simulink model "E040S1_R2_transfer_drain_iqcot_20260630"  (R2024b)
settings: Solver=VariableStepAuto  StartTime=0.0  StopTime=0.52e-3  MaxStep=5e-9  RelTol=1e-3
undefined symbols (not defined in the file): A_init, A_lower, A_upper, Cout, DCR_L1, DCR_L2, DCR_L3, DCR_L4, E040_Calibration_Enable, E040_Current_Deadband, E040_Current_Limit_A, E040_Disabled_Phase_Drain_Timeout, E040_Dwell_Time, E040_Fallback_K_T, E040_I_Shed_Low, E040_IL_Sense_Gain1, E040_IL_Sense_Gain2, E040_IL_Sense_Gain3, E040_IL_Sense_Gain4, E040_K_T, E040_LoadStep_Time, E040_Max_Transfer_Ton_Trim, E040_Min_Scale, E040_Order_Relock_Window, E040_Post_Reentry_Shed_Delay, E040_Post_Shed_AS_Delay, E040_Remaining_Phase_Current_Limit, E040_Residual_Current_Threshold, E040_Sense_Confidence, E040_Severe_Overshoot_Band, E040_Shed_Commit_Boundary_Policy, E040_Shed_Fallback_Enable, E040_Shed_Transfer_Rate, E040_Shed_Transfer_Window, E040_Shed_Undershoot_Budget, E040_T_Trim_Max, E040_TonDiff_Enable, E040_V_Error_Budget, E040_V_Error_Hard_Limit, E040_Variant_Mode, E040_Vref, ESR_C, IdealIQCOT_Enable, IL_adc_counts_per_A, IL_pk_limit_adc_neg, IL_pk_limit_adc_pos, Iload_final, Iload_initial, Iph, Iqcot_enable, kappa_cmd, Kiqcot, Kvc_iqcot, L, Lambda0_iqcot, Lambda_m2, rho_cmd, Ri_iqcot, t_load_step, Tblank ... (+15)
libraries: simulink x29, spsCurrentMeasurementLib x8, spsMosfetLib x8, spsSeriesRLCBranchLib x5, spsVoltageMeasurementLib x5, spsDCVoltageSourceLib x4, spsControlledCurrentSourceLib x1, spsGroundLib x1, spspowerguiLib x1
(part 2 of 2)

== system E040S1_R2_transfer_drain_iqcot_20260630/OnDelay ==
  u : Inport
  Compare To Constant : simulink/Logic and Bit Operations/Compare To Constant  relop=>=  const=Tdead  OutDataTypeStr=boolean
  Data Type Conversion : DataTypeConversion  OutDataTypeStr=double  SaturateOnIntegerOverflow=off  RndMeth=Floor
  Integrator : Integrator  ExternalReset=level
  Logical Operator : Logic  Operator=NOT  AllPortsSameDT=off  OutDataTypeStr=boolean
  y : Outport
  wires:
  u/1 -> Data Type Conversion/1, Logical Operator/1
  Logical Operator/1 -> Integrator/2
  Data Type Conversion/1 -> Integrator/1
  Integrator/1 -> Compare To Constant/1
  Compare To Constant/1 -> y/1

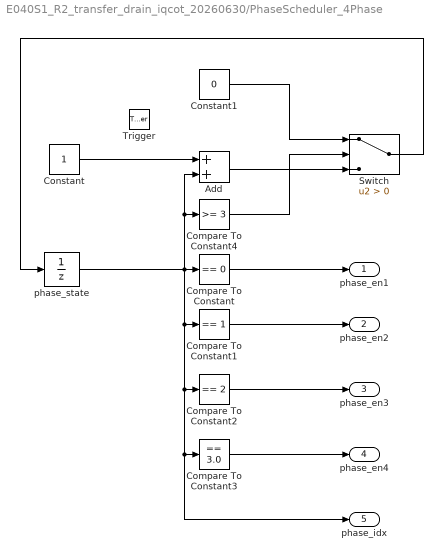
== system E040S1_R2_transfer_drain_iqcot_20260630/PhaseScheduler_4Phase ==
  Trigger : TriggerPort  VariantControl=(inherit)
  Add : Sum
  Compare To Constant : simulink/Logic and Bit Operations/Compare To Constant  relop===  const=0  OutDataTypeStr=boolean
  Compare To Constant1 : simulink/Logic and Bit Operations/Compare To Constant  relop===  const=1  OutDataTypeStr=boolean
  Compare To Constant2 : simulink/Logic and Bit Operations/Compare To Constant  relop===  const=2  OutDataTypeStr=boolean
  Compare To Constant3 : simulink/Logic and Bit Operations/Compare To Constant  relop===  const=3.0  OutDataTypeStr=boolean
  Compare To Constant4 : simulink/Logic and Bit Operations/Compare To Constant  relop=>=  const=3  OutDataTypeStr=boolean
  Constant : Constant
  Constant1 : Constant  Value=0
  Switch : Switch  Criteria=u2 > Threshold  SaturateOnIntegerOverflow=off  InputSameDT=off
  phase_state : UnitDelay  SampleTime=-1  HasFrameUpgradeWarning=on
  phase_en1 : Outport
  phase_en2 : Outport  Port=2
  phase_en3 : Outport  Port=3
  phase_en4 : Outport  Port=4
  phase_idx : Outport  Port=5
  wires:
  phase_state/1 -> phase_idx/1, Compare To Constant3/1, Compare To Constant2/1, Compare To Constant1/1, Compare To Constant/1, Compare To Constant4/1, Add/2
  Compare To Constant/1 -> phase_en1/1
  Compare To Constant1/1 -> phase_en2/1
  Compare To Constant2/1 -> phase_en3/1
  Compare To Constant3/1 -> phase_en4/1
  Constant/1 -> Add/1
  Add/1 -> Switch/3
  Compare To Constant4/1 -> Switch/2
  Constant1/1 -> Switch/1
  Switch/1 -> phase_state/1

== system E040S1_R2_transfer_drain_iqcot_20260630/GateDriver_1Phase1/OnDelay ==
  u : Inport
  Compare To Constant : simulink/Logic and Bit Operations/Compare To Constant  relop=>=  const=Tdead  OutDataTypeStr=boolean
  Data Type Conversion : DataTypeConversion  OutDataTypeStr=double  SaturateOnIntegerOverflow=off  RndMeth=Floor
  Integrator : Integrator  ExternalReset=level
  Logical Operator : Logic  Operator=NOT  AllPortsSameDT=off  OutDataTypeStr=boolean
  y : Outport
  wires:
  u/1 -> Data Type Conversion/1, Logical Operator/1
  Logical Operator/1 -> Integrator/2
  Data Type Conversion/1 -> Integrator/1
  Integrator/1 -> Compare To Constant/1
  Compare To Constant/1 -> y/1

== system E040S1_R2_transfer_drain_iqcot_20260630/GateDriver_1Phase1/OnDelay1 ==
  u : Inport
  Compare To Constant : simulink/Logic and Bit Operations/Compare To Constant  relop=>=  const=Tdead  OutDataTypeStr=boolean
  Data Type Conversion : DataTypeConversion  OutDataTypeStr=double  SaturateOnIntegerOverflow=off  RndMeth=Floor
  Integrator : Integrator  ExternalReset=level
  Logical Operator : Logic  Operator=NOT  AllPortsSameDT=off  OutDataTypeStr=boolean
  y : Outport
  wires:
  u/1 -> Data Type Conversion/1, Logical Operator/1
  Logical Operator/1 -> Integrator/2
  Data Type Conversion/1 -> Integrator/1
  Integrator/1 -> Compare To Constant/1
  Compare To Constant/1 -> y/1

== system E040S1_R2_transfer_drain_iqcot_20260630/GateDriver_1Phase2/OnDelay ==
  u : Inport
  Compare To Constant : simulink/Logic and Bit Operations/Compare To Constant  relop=>=  const=Tdead  OutDataTypeStr=boolean
  Data Type Conversion : DataTypeConversion  OutDataTypeStr=double  SaturateOnIntegerOverflow=off  RndMeth=Floor
  Integrator : Integrator  ExternalReset=level
  Logical Operator : Logic  Operator=NOT  AllPortsSameDT=off  OutDataTypeStr=boolean
  y : Outport
  wires:
  u/1 -> Data Type Conversion/1, Logical Operator/1
  Logical Operator/1 -> Integrator/2
  Data Type Conversion/1 -> Integrator/1
  Integrator/1 -> Compare To Constant/1
  Compare To Constant/1 -> y/1

== system E040S1_R2_transfer_drain_iqcot_20260630/GateDriver_1Phase2/OnDelay1 ==
  u : Inport
  Compare To Constant : simulink/Logic and Bit Operations/Compare To Constant  relop=>=  const=Tdead  OutDataTypeStr=boolean
  Data Type Conversion : DataTypeConversion  OutDataTypeStr=double  SaturateOnIntegerOverflow=off  RndMeth=Floor
  Integrator : Integrator  ExternalReset=level
  Logical Operator : Logic  Operator=NOT  AllPortsSameDT=off  OutDataTypeStr=boolean
  y : Outport
  wires:
  u/1 -> Data Type Conversion/1, Logical Operator/1
  Logical Operator/1 -> Integrator/2
  Data Type Conversion/1 -> Integrator/1
  Integrator/1 -> Compare To Constant/1
  Compare To Constant/1 -> y/1

== system E040S1_R2_transfer_drain_iqcot_20260630/GateDriver_1Phase3/OnDelay ==
  u : Inport
  Compare To Constant : simulink/Logic and Bit Operations/Compare To Constant  relop=>=  const=Tdead  OutDataTypeStr=boolean
  Data Type Conversion : DataTypeConversion  OutDataTypeStr=double  SaturateOnIntegerOverflow=off  RndMeth=Floor
  Integrator : Integrator  ExternalReset=level
  Logical Operator : Logic  Operator=NOT  AllPortsSameDT=off  OutDataTypeStr=boolean
  y : Outport
  wires:
  u/1 -> Data Type Conversion/1, Logical Operator/1
  Logical Operator/1 -> Integrator/2
  Data Type Conversion/1 -> Integrator/1
  Integrator/1 -> Compare To Constant/1
  Compare To Constant/1 -> y/1

== system E040S1_R2_transfer_drain_iqcot_20260630/GateDriver_1Phase3/OnDelay1 ==
  u : Inport
  Compare To Constant : simulink/Logic and Bit Operations/Compare To Constant  relop=>=  const=Tdead  OutDataTypeStr=boolean
  Data Type Conversion : DataTypeConversion  OutDataTypeStr=double  SaturateOnIntegerOverflow=off  RndMeth=Floor
  Integrator : Integrator  ExternalReset=level
  Logical Operator : Logic  Operator=NOT  AllPortsSameDT=off  OutDataTypeStr=boolean
  y : Outport
  wires:
  u/1 -> Data Type Conversion/1, Logical Operator/1
  Logical Operator/1 -> Integrator/2
  Data Type Conversion/1 -> Integrator/1
  Integrator/1 -> Compare To Constant/1
  Compare To Constant/1 -> y/1

== system E040S1_R2_transfer_drain_iqcot_20260630/GateDriver_1Phase4/OnDelay ==
  u : Inport
  Compare To Constant : simulink/Logic and Bit Operations/Compare To Constant  relop=>=  const=Tdead  OutDataTypeStr=boolean
  Data Type Conversion : DataTypeConversion  OutDataTypeStr=double  SaturateOnIntegerOverflow=off  RndMeth=Floor
  Integrator : Integrator  ExternalReset=level
  Logical Operator : Logic  Operator=NOT  AllPortsSameDT=off  OutDataTypeStr=boolean
  y : Outport
  wires:
  u/1 -> Data Type Conversion/1, Logical Operator/1
  Logical Operator/1 -> Integrator/2
  Data Type Conversion/1 -> Integrator/1
  Integrator/1 -> Compare To Constant/1
  Compare To Constant/1 -> y/1

== system E040S1_R2_transfer_drain_iqcot_20260630/GateDriver_1Phase4/OnDelay1 ==
  u : Inport
  Compare To Constant : simulink/Logic and Bit Operations/Compare To Constant  relop=>=  const=Tdead  OutDataTypeStr=boolean
  Data Type Conversion : DataTypeConversion  OutDataTypeStr=double  SaturateOnIntegerOverflow=off  RndMeth=Floor
  Integrator : Integrator  ExternalReset=level
  Logical Operator : Logic  Operator=NOT  AllPortsSameDT=off  OutDataTypeStr=boolean
  y : Outport
  wires:
  u/1 -> Data Type Conversion/1, Logical Operator/1
  Logical Operator/1 -> Integrator/2
  Data Type Conversion/1 -> Integrator/1
  Integrator/1 -> Compare To Constant/1
  Compare To Constant/1 -> y/1

== matlab function E040S1_R2_transfer_drain_iqcot_20260630/E040_S1_StagedShedSupervisor ==
  data: req1 input boolean; req1o output boolean; req2 input boolean; req3 input boolean; req4 input boolean; ton1 input double; ton2 input double; ton3 input double; ton4 input double; il1 input double; il2 input double; il3 input double; il4 input double; vout input double; iload input double; t input double; t_step input double; variant_mode input double; I_shed_low input double; dwell_time input double; post_reentry_shed_delay input double; Vref input double; severe_overshoot_band input double; current_limit_A input double; TonDiff_enable input double; K_T input double; fallback_K_T input double; T_trim_Max input double; current_deadband input double; sense_confidence input double; calibration_enable input double; Verr_budget input double; Verr_hard input double; min_scale input double; residual_current_threshold input double; order_relock_window input double; shed_transfer_rate input double; shed_transfer_window input double; max_transfer_Ton_trim input double; remaining_phase_current_limit_guard input double; disabled_phase_drain_timeout input double; shed_undershoot_budget input double; post_shed_aS_delay input double; shed_fallback_enable input double; shed_commit_boundary_policy input double; req2o output boolean; req3o output boolean; req4o output boolean; ton1o output double; ton2o output double; ton3o output double; ton4o output double; active_phase_set output double; N_active output double; phase_shed_request output double; phase_shed_accept output double; phase_shed_reject output double; phase_add_request output double; shed_state output double; shed_lockout_state output double; residual_current_i output double; residual_current_threshold_o output double; residual_current_check output double; dwell_timer output double; post_reentry_shed_delay_timer output double; protect_state output double; reentry_state output double; balance_recovery_state output double; sense_confidence_o output double; calibration_enable_o output double; a_S_mode output double; fallback_count_o output double; guard_clamp_count_o output double; trim1 output double; trim2 output double; trim3 output double; trim4 output double; REQ_accept1 output boolean; REQ_accept2 output boolean; REQ_accept3 output boolean; REQ_accept4 output boolean; REQ_reject_reason output double; logical_slot output double; physical_phase_selected output double; phase_shed_reject_reason output double; order_relock_state output double; order_relock_window_done output double; phase_order_error_rate_window output double; a_S_enable_after_shed output double; current_limit_hit output double; shed_transfer_progress output double; disabled_phase_current_sum output double; commit_armed output double; commit_done output double; shed_commit_count output double; fallback_4ph_triggered output double; fallback_reason output double; fallback_4ph_count output double; residual_current_phase2_A output double; residual_current_phase4_A output double; Ton_trim_usage output double; Lambda_trim_usage output double; phase_gate_enable1 output double; phase_gate_enable2 output double; phase_gate_enable3 output double; phase_gate_enable4 output double
function [req1o,req2o,req3o,req4o,ton1o,ton2o,ton3o,ton4o,active_phase_set,N_active,phase_shed_request,phase_shed_accept,phase_shed_reject,phase_add_request,shed_state,shed_lockout_state,residual_current_i,residual_current_threshold_o,residual_current_check,dwell_timer,post_reentry_shed_delay_timer,protect_state,reentry_state,balance_recovery_state,sense_confidence_o,calibration_enable_o,a_S_mode,fallback_count_o,guard_clamp_count_o,trim1,trim2,trim3,trim4,REQ_accept1,REQ_accept2,REQ_accept3,REQ_accept4,REQ_reject_reason,logical_slot,physical_phase_selected,phase_shed_reject_reason,order_relock_state,order_relock_window_done,phase_order_error_rate_window,a_S_enable_after_shed,current_limit_hit,shed_transfer_progress,disabled_phase_current_sum,commit_armed,commit_done,shed_commit_count,fallback_4ph_triggered,fallback_reason,fallback_4ph_count,residual_current_phase2_A,residual_current_phase4_A,Ton_trim_usage,Lambda_trim_usage,phase_gate_enable1,phase_gate_enable2,phase_gate_enable3,phase_gate_enable4] = e040_s1_supervisor(req1,req2,req3,req4,ton1,ton2,ton3,ton4,il1,il2,il3,il4,vout,iload,t,t_step,variant_mode,I_shed_low,dwell_time,post_reentry_shed_delay,Vref,severe_overshoot_band,current_limit_A,TonDiff_enable,K_T,fallback_K_T,T_trim_Max,current_deadband,sense_confidence,calibration_enable,Verr_budget,Verr_hard,min_scale,residual_current_threshold,order_relock_window,shed_transfer_rate,shed_transfer_window,max_transfer_Ton_trim,remaining_phase_current_limit_guard,disabled_phase_drain_timeout,shed_undershoot_budget,post_shed_aS_delay,shed_fallback_enable,shed_commit_boundary_policy)
%#codegen
req = [req1, req2, req3, req4] > 0.5;
tons = [ton1, ton2, ton3, ton4];
ils = [il1, il2, il3, il4];
phase_add_request = 0.0;
protect_state = 0.0;
reentry_state = 1.0;
sense_confidence_o = sense_confidence;
calibration_enable_o = calibration_enable;
residual_current_threshold_o = residual_current_threshold;
residual_current_phase2_A = il2;
residual_current_phase4_A = il4;
residual_current_i = [0.0, il2, 0.0, il4];
disabled_phase_current_sum = abs(il2) + abs(il4);
residual_ok = (residual_current_threshold > 0.0) && (abs(il2) <= residual_current_threshold) && (abs(il4) <= residual_current_threshold);
residual_current_check = double(residual_ok);
age = max(0.0, t - t_step);
request_active = (variant_mode > 0.5) && (iload < I_shed_low) && (t >= t_step);
phase_shed_request = double(request_active);
if request_active
    dwell_timer = age;
    post_reentry_shed_delay_timer = age;
else
    dwell_timer = 0.0;
    post_reentry_shed_delay_timer = 0.0;
end
transfer_window = max(shed_transfer_window, 1.0e-9);
drain_timeout = max(disabled_phase_drain_timeout, 0.0);
drain_deadline_age = transfer_window + drain_timeout;
post_transfer_age = max(0.0, age - transfer_window);
shed_transfer_progress = 0.0;
if request_active
    shed_transfer_progress = min(max(age / transfer_window, 0.0), 1.0);
end
phase2_drained = request_active && (variant_mode >= 2.0) && (shed_transfer_progress >= 0.5) && (residual_current_threshold > 0.0) && (abs(il2) <= residual_current_threshold);
phase4_drained = request_active && (variant_mode >= 2.0) && (shed_transfer_progress >= 0.5) && (residual_current_threshold > 0.0) && (abs(il4) <= residual_current_threshold);
current_limit_hit = double((current_limit_A > 0.0) && (max(abs(ils)) >= current_limit_A));
remaining_peak = max(abs(il1), abs(il3));
remaining_headroom_ok = (remaining_phase_current_limit_guard <= 0.0) || (remaining_peak < remaining_phase_current_limit_guard);
voltage_ok = (vout >= (Vref - shed_undershoot_budget)) && (vout <= (Vref + severe_overshoot_band));
drain_time_ok = (drain_timeout <= 0.0) || (age <= drain_deadline_age);
drain_timeout_fail = request_active && (variant_mode >= 3.0) && (age > drain_deadline_age) && ~residual_ok;
hard_guard_fail = request_active && (shed_fallback_enable > 0.5) && ((vout < Vref - shed_undershoot_budget) || current_limit_hit > 0.5 || ~remaining_headroom_ok || drain_timeout_fail);
fallback_4ph_triggered = double(hard_guard_fail);
fallback_4ph_count = fallback_4ph_triggered;
fallback_count_o = fallback_4ph_triggered;
fallback_reason = 0.0;
if hard_guard_fail
    if vout < Vref - shed_undershoot_budget
        fallback_reason = 1.0;
    elseif current_limit_hit > 0.5
        fallback_reason = 2.0;
    elseif drain_timeout_fail
        fallback_reason = 3.0;
    elseif ~remaining_headroom_ok
        fallback_reason = 5.0;
    else
        fallback_reason = 6.0;
    end
end
immediate_shed = request_active && (variant_mode >= 1.0) && (variant_mode < 2.0);
allow_commit_variant = variant_mode >= 3.0;
commit_ready = request_active && allow_commit_variant && (age >= transfer_window) && residual_ok && remaining_headroom_ok && voltage_ok && drain_time_ok && ~hard_guard_fail;
commit_hold = request_active && allow_commit_variant && (age >= transfer_window) && remaining_headroom_ok && voltage_ok && ~hard_guard_fail;
commit_armed = double(commit_ready || commit_hold || immediate_shed);
commit_done = double(commit_hold || immediate_shed);
shed_commit_count = commit_done;
commit_age = post_transfer_age;
order_relock_done = (commit_done > 0.5) && (commit_age >= max(order_relock_window, 0.0));
order_relock_window_done = double(order_relock_done);
a_S_enable_after_shed = double((variant_mode >= 4.0) && (TonDiff_enable > 0.5) && (commit_done > 0.5) && order_relock_done && residual_ok && voltage_ok && (commit_age >= max(post_shed_aS_delay, 0.0)));
balance_enable = a_S_enable_after_shed > 0.5;
phase_shed_accept = commit_done;
phase_shed_reject = double(request_active && commit_done < 0.5);
phase_shed_reject_reason = 0.0;
if phase_shed_reject > 0.5
    if hard_guard_fail
        phase_shed_reject_reason = fallback_reason;
    elseif age < transfer_window
        phase_shed_reject_reason = 2.0;
    elseif ~residual_ok
        phase_shed_reject_reason = 3.0;
    elseif ~remaining_headroom_ok
        phase_shed_reject_reason = 5.0;
    else
        phase_shed_reject_reason = 1.0;
    end
end
if ~request_active
    shed_state = 0.0;
    shed_lockout_state = 0.0;
    order_relock_state = 0.0;
elseif hard_guard_fail
    shed_state = 9.0;
    shed_lockout_state = 1.0;
    order_relock_state = 0.0;
elseif age < 1.0e-7
    shed_state = 1.0;
    shed_lockout_state = 0.0;
    order_relock_state = 1.0;
elseif age < transfer_window
    shed_state = 2.0;
    shed_lockout_state = 0.0;
    order_relock_state = 1.0;
elseif immediate_shed
    shed_state = 5.0;
    shed_lockout_state = 0.0;
    order_relock_state = 2.0;
elseif age >= transfer_window && (~residual_ok || ~remaining_headroom_ok || ~voltage_ok)
    shed_state = 3.0;
    shed_lockout_state = 0.0;
    order_relock_state = 1.0;
elseif variant_mode < 3.0
    shed_state = 3.0;
    shed_lockout_state = 0.0;
    order_relock_state = 1.0;
elseif commit_done < 0.5
    shed_state = 4.0;
    shed_lockout_state = 0.0;
    order_relock_state = 1.0;
elseif commit_age < 5.0e-8
    shed_state = 5.0;
    shed_lockout_state = 0.0;
    order_relock_state = 2.0;
elseif ~order_relock_done
    shed_state = 6.0;
    shed_lockout_state = 0.0;
    order_relock_state = 2.0;
elseif balance_enable
    shed_state = 7.0;
    shed_lockout_state = 0.0;
    order_relock_state = 3.0;
else
    shed_state = 8.0;
    shed_lockout_state = 0.0;
    order_relock_state = 3.0;
end
trim = [0.0, 0.0, 0.0, 0.0];
if request_active && ~hard_guard_fail && (variant_mode >= 2.0) && (commit_done < 0.5)
    p = shed_transfer_progress;
    transfer_trim = min(max_transfer_Ton_trim, T_trim_Max);
    if transfer_trim < 0.0
        transfer_trim = 0.0;
    end
    trim = [p * transfer_trim, -p * transfer_trim, p * transfer_trim, -p * transfer_trim];
end
REQ_reject_reason = 0.0;
if hard_guard_fail
    active_phase_set = [1.0, 1.0, 1.0, 1.0];
    N_active = 4.0;
    req_out = req;
    ton_base = tons;
elseif commit_done > 0.5
    active_phase_set = [1.0, 0.0, 1.0, 0.0];
    N_active = 2.0;
    req_out = [req(1) || req(3), false, req(2) || req(4), false];
    ton_base = [ton1, 0.0, ton3, 0.0];
elseif request_active && (variant_mode >= 2.0) && (age >= transfer_window)
    active_phase_set = [1.0, 1.0, 1.0, 1.0];
    N_active = 4.0;
    req_out = [req(1) || req(3), false, req(2) || req(4), false];
    ton_base = [ton1, 0.0, ton3, 0.0];
elseif request_active && (variant_mode >= 2.0) && (phase2_drained || phase4_drained)
    active_phase_set = [1.0, 1.0, 1.0, 1.0];
    N_active = 4.0;
    req_out = req;
    ton_base = tons;
    if phase2_drained
        req_out(3) = req_out(3) || req(2);
        req_out(2) = false;
        ton_base(2) = 0.0;
    end
    if phase4_drained
        req_out(3) = req_out(3) || req(4);
        req_out(4) = false;
        ton_base(4) = 0.0;
    end
else
    active_phase_set = [1.0, 1.0, 1.0, 1.0];
    N_active = 4.0;
    req_out = req;
    ton_base = tons;
end
if any(req) && ~any(req_out) && REQ_reject_reason == 0.0
    REQ_reject_reason = 1.0;
end
if req_out(1)
    logical_slot = 1.0; physical_phase_selected = 1.0;
elseif req_out(2)
    logical_slot = 2.0; physical_phase_selected = 2.0;
elseif req_out(3)
    if commit_done > 0.5
        logical_slot = 2.0;
    else
        logical_slot = 3.0;
    end
    physical_phase_selected = 3.0;
elseif req_out(4)
    logical_slot = 4.0; physical_phase_selected = 4.0;
else
    logical_slot = 0.0; physical_phase_selected = 0.0;
end
a_S_mode = 0.0;
guard_clamp = 0.0;
if balance_enable
    active_mask = active_phase_set > 0.5;
    K_eff = fallback_K_T;
    a_S_mode = 1.0;
    denom = max(sum(double(active_mask)), 1.0);
    avg_i = sum(ils .* double(active_mask)) / denom;
    err = (ils - avg_i) .* double(active_mask);
    raw = -K_eff .* err;
    if max(abs(err)) < current_deadband
        raw = [0.0, 0.0, 0.0, 0.0];
    end
    trim_as = min(max(raw, -T_trim_Max), T_trim_Max);
    trim_mean = sum(trim_as .* double(active_mask)) / denom;
    trim_as = (trim_as - trim_mean) .* double(active_mask);
    trim = trim + trim_as;
end
ton_out = max([0.0, 0.0, 0.0, 0.0], ton_base + trim);
phase_order_error_rate_window = 0.0;
balance_recovery_state = double(balance_enable);
Ton_trim_usage = 0.0;
if T_trim_Max > 0.0
    Ton_trim_usage = max(abs(trim)) / T_trim_Max;
end
Lambda_trim_usage = 0.0;
gate_enable = [1.0, 1.0, 1.0, 1.0];
if phase2_drained
    gate_enable(2) = 0.0;
end
if phase4_drained
    gate_enable(4) = 0.0;
end
if (commit_done > 0.5) || immediate_shed
    gate_enable = [1.0, 0.0, 1.0, 0.0];
end
if hard_guard_fail
    gate_enable = [1.0, 1.0, 1.0, 1.0];
end
req1o = req_out(1); req2o = req_out(2); req3o = req_out(3); req4o = req_out(4);
ton1o = ton_out(1); ton2o = ton_out(2); ton3o = ton_out(3); ton4o = ton_out(4);
guard_clamp_count_o = guard_clamp;
trim1 = trim(1); trim2 = trim(2); trim3 = trim(3); trim4 = trim(4);
REQ_accept1 = req_out(1); REQ_accept2 = req_out(2); REQ_accept3 = req_out(3); REQ_accept4 = req_out(4);
phase_gate_enable1 = gate_enable(1); phase_gate_enable2 = gate_enable(2); phase_gate_enable3 = gate_enable(3); phase_gate_enable4 = gate_enable(4);

== matlab function E040S1_R2_transfer_drain_iqcot_20260630/Ideal_Digital_IQCOT_Request/IQCOT_Event_Core ==
  data: e_v input double size=1; REQ_iqcot output double size=1; IL1 input double size=1; IL2 input double size=1; IL3 input double size=1; IL4 input double size=1; phase_idx input double size=1; tr_reset input double size=1; enable input double size=1; Ts_ctrl_in input double size=1; Lambda0_in input double size=1; Lambda_m2_in input double size=1; rho_cmd_in input double size=1; Ri_in input double size=1; Kvc_in input double size=1; Vc_bias_in input double size=1; kappa_cmd_in input double size=1; A_init_in input double size=1; A_lower_in input double size=1; A_upper_in input double size=1; A_iqcot output double size=1; Lambda_i output double size=1; h_iqcot output double size=1; IL_sel output double size=1; vc_ctrl output double size=1
function [REQ_iqcot,A_iqcot,Lambda_i,h_iqcot,IL_sel,vc_ctrl] = IQCOT_Event_Core(e_v,IL1,IL2,IL3,IL4,phase_idx,tr_reset,enable,Ts_ctrl_in,Lambda0_in,Lambda_m2_in,rho_cmd_in,Ri_in,Kvc_in,Vc_bias_in,kappa_cmd_in,A_init_in,A_lower_in,A_upper_in)
%#codegen
REQ_iqcot = 0.0;
A_iqcot = 0.0;
Lambda_i = 0.0;
h_iqcot = 0.0;
IL_sel = 0.0;
vc_ctrl = 0.0;
persistent Astate reset_prev phase_prev
if isempty(Astate)
    Astate = double(A_init_in);
end
if isempty(reset_prev)
    reset_prev = 0.0;
end
if isempty(phase_prev)
    phase_prev = 0.0;
end
p = floor(double(phase_idx));
p = mod(p, 4);
if p == 0
    IL_sel = IL1;
elseif p == 1
    IL_sel = IL2;
elseif p == 2
    IL_sel = IL3;
else
    IL_sel = IL4;
end
Ri_eff = Ri_in * exp(kappa_cmd_in);
vc_ctrl = Vc_bias_in + Kvc_in * e_v;
h_iqcot = vc_ctrl - Ri_eff * IL_sel;
Lambda_i = Lambda0_in * (1 + rho_cmd_in) + Lambda_m2_in * cos(pi * p);
if Lambda_i < eps
    Lambda_i = eps;
end
A_update = Astate + Ts_ctrl_in * h_iqcot;
if A_update < A_lower_in
    A_update = A_lower_in;
end
if A_update > A_upper_in
    A_update = A_upper_in;
end
REQ_iqcot = double((enable > 0.5) && (A_update >= Lambda_i));
A_iqcot = A_update;
reset_rise = (tr_reset > 0.5) && (reset_prev <= 0.5);
phase_change = (p ~= phase_prev);
if enable <= 0.5
    Astate = A_init_in;
elseif reset_rise || phase_change
    Astate = A_init_in;
else
    Astate = A_update;
end
reset_prev = double(tr_reset);
phase_prev = p;

== matlab function E040S1_R2_transfer_drain_iqcot_20260630/E040_TonActual1 ==
  data: qh input boolean; Ton_actual output double; t input double
function Ton_actual = ton_actual_estimator(qh, t)
%#codegen
persistent q_prev t_rise last_width
if isempty(q_prev)
    q_prev = 0.0;
end
if isempty(t_rise)
    t_rise = 0.0;
end
if isempty(last_width)
    last_width = 0.0;
end
is_high = double(qh > 0.5);
if is_high > 0.5 && q_prev <= 0.5
    t_rise = t;
elseif is_high <= 0.5 && q_prev > 0.5
    last_width = max(0.0, t - t_rise);
end
Ton_actual = last_width;
q_prev = is_high;

== matlab function E040S1_R2_transfer_drain_iqcot_20260630/E040_TonActual2 ==
  data: qh input boolean; Ton_actual output double; t input double
function Ton_actual = ton_actual_estimator(qh, t)
%#codegen
persistent q_prev t_rise last_width
if isempty(q_prev)
    q_prev = 0.0;
end
if isempty(t_rise)
    t_rise = 0.0;
end
if isempty(last_width)
    last_width = 0.0;
end
is_high = double(qh > 0.5);
if is_high > 0.5 && q_prev <= 0.5
    t_rise = t;
elseif is_high <= 0.5 && q_prev > 0.5
    last_width = max(0.0, t - t_rise);
end
Ton_actual = last_width;
q_prev = is_high;

== matlab function E040S1_R2_transfer_drain_iqcot_20260630/E040_TonActual3 ==
  data: qh input boolean; Ton_actual output double; t input double
function Ton_actual = ton_actual_estimator(qh, t)
%#codegen
persistent q_prev t_rise last_width
if isempty(q_prev)
    q_prev = 0.0;
end
if isempty(t_rise)
    t_rise = 0.0;
end
if isempty(last_width)
    last_width = 0.0;
end
is_high = double(qh > 0.5);
if is_high > 0.5 && q_prev <= 0.5
    t_rise = t;
elseif is_high <= 0.5 && q_prev > 0.5
    last_width = max(0.0, t - t_rise);
end
Ton_actual = last_width;
q_prev = is_high;

== matlab function E040S1_R2_transfer_drain_iqcot_20260630/E040_TonActual4 ==
  data: qh input boolean; Ton_actual output double; t input double
function Ton_actual = ton_actual_estimator(qh, t)
%#codegen
persistent q_prev t_rise last_width
if isempty(q_prev)
    q_prev = 0.0;
end
if isempty(t_rise)
    t_rise = 0.0;
end
if isempty(last_width)
    last_width = 0.0;
end
is_high = double(qh > 0.5);
if is_high > 0.5 && q_prev <= 0.5
    t_rise = t;
elseif is_high <= 0.5 && q_prev > 0.5
    last_width = max(0.0, t - t_rise);
end
Ton_actual = last_width;
q_prev = is_high;
